simulink model "nlmodel"  (Simulink 4.00)
settings: Solver=ode45  StartTime=0.0  StopTime=10.0  RelTol=1e-3
values from neighbouring files (symbols this model uses):
  x0 = [2;0]    [linid.m]    (also in nonlinid.m = [0;0]; sfdcmotorin.m = []; sfdcmotorout.m = [])
undefined symbols (not defined in the file or in its folder): bhat
settings Model: LastModifiedBy=R.Babuska

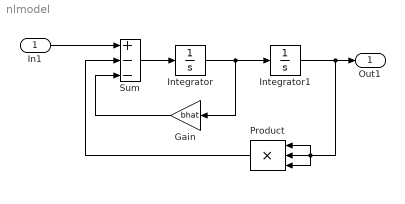
== system nlmodel ==
  In1 : Inport  Port=1  LatchInput=off
  Gain : Gain  Orientation=left  Gain=bhat  Multiplication=Element-wise(K.*u)  SaturateOnIntegerOverflow=on
  Integrator : Integrator  ExternalReset=none  InitialConditionSource=internal  InitialCondition=x0(2)  LimitOutput=off  UpperSaturationLimit=inf  LowerSaturationLimit=-inf  ShowSaturationPort=off  ShowStatePort=off  AbsoluteTolerance=auto
  Integrator1 : Integrator  ExternalReset=none  InitialConditionSource=internal  InitialCondition=x0(1)  LimitOutput=off  UpperSaturationLimit=inf  LowerSaturationLimit=-inf  ShowSaturationPort=off  ShowStatePort=off  AbsoluteTolerance=auto
  Product : Product  Orientation=left  Inputs=3  Multiplication=Element-wise(.*)  SaturateOnIntegerOverflow=on
  Sum : Sum  Inputs=+--  SaturateOnIntegerOverflow=on
  Out1 : Outport  Port=1
  wires:
  Integrator/1 -> Integrator1/1, Gain/1
  Sum/1 -> Integrator/1
  Integrator1/1 -> Product/2, Product/1, Product/3, Out1/1
  Product/1 -> Sum/2
  Gain/1 -> Sum/3
  In1/1 -> Sum/1
